simulink model "example6"  (Simulink 7.1)
settings: Solver=ode45  StartTime=0.0  StopTime=10.0  MaxStep=0.1  RelTol=1e-3
model workspace: external: M-Code (data not in the file)
undefined symbols (not defined in the file): doubleElbow, FDgq, J
libraries: simulink x5
settings Model: Creator=roy  LastModifiedBy=roy
settings DataIOCC: LimitDataPoints=off

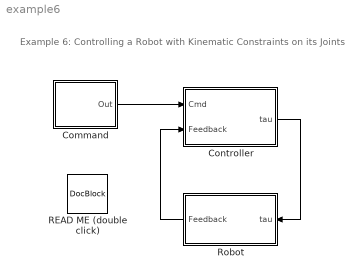
== system example6 ==
  note: Example 6: Controlling a Robot with
      | Kinematic Constraints on its Joints
  Command : Subsystem
  Controller : Subsystem
  READ ME (double click) : simulink/Model-Wide Utilities/DocBlock  SystemSampleTime=-1  DocumentType=Text
      content=|
      | This Simulink model follows on from Example 1 (with organizational
      | elements from Example 2), in which a simple PD control law was used to
      | control the motion of a planar 2R robot mechanism.  The new feature in
      | this example is that the robot is subject to a kinematic constraint on its
      | joint variables.
      |
      | Specifically, the robot in this example is a modification of the planar 2R
      | mechanism in which the elbow joint has been replaced by a pair of revolute
      | joints close together, which are subject to a 1:1 gearing constraint
      | (i.e., the two joint variables are constrained to be the same).  This is
      | the kind of joint one gets from two equal-radius cylinders rolling over
      | each other without slipping.  The robot therefore has three joint
      | variables in total, but q(2) is constrained to be equal to q(3).
      |
      | There is also a new feature to be found in the control system.  The
      | controller is interested in controlling this robot as if the elbow were a
      | single compound joint with a single joint variable.  Therefore, the
      | controller seeks to control the two variables q(1) and q(2)+q(3), the
      | latter being the angle between the two main links in the mechanism; and
      | the signal generated by the command subsystem consists of a commanded
      | value for q(1) and a commanded value for q(2)+q(3).  The controller
      | subsystem therefore contains extra blocks that translate from the
      | mechanism's joint space to the control system's command space and back
      | again.  For more details, see the controller subsystem's documantation
      | block.
      |
      | The dynamics calculation for a mechanism with kinematic constraints among
      | its joint variables is performed by FDgq.  This function expects to find a
      | field called "gamma_q" in the model data structure, containing the handle
      | of a function that formulates the constraint equations.  FDgq then solves
      | the equation of motion in a manner that complies with the constraints.
      | More details can be found in the documentation block in the robot
      | subsystem.
      |
      | If you run this simulation, then you will immediately see that the
      | controller is badly tuned, just like in Example 1, so you can see the
      | dynamics in action.  It is particularly obvious that the wobbling when the
      | robot is straight is at a lower frequency, and is less damped, than the
      | wobbling when the robot is bent.  Adjusting the gains (in particular,
      | higher gains for joint 1) will improve the performance.  In contrast to
      | the poor tracking accuracy of the control system, the kinematic constraint
      | on q(2) and q(3) is maintained exactly.
      |
      | To view the motion with showmotion, use the command
      | "showmotion(doubleElbow,tout,qout)".
  Robot : Subsystem  Orientation=left
  wires:
  Command/1(Out) -> Controller/1(Cmd)
  Robot/1(Feedback) -> Controller/2(Feedback)
  Controller/1(tau) -> Robot/1(tau)

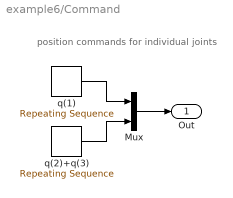
== system example6/Command ==
  note: position commands for
      | individual joints
  Mux : Mux  Inputs=2
  q(1) : simulink/Sources/Repeating Sequence  SystemSampleTime=-1  rep_seq_t=[0 1 2 3 4]  rep_seq_y=[0 1 1 0 0]
  q(2)+q(3) : simulink/Sources/Repeating Sequence  SystemSampleTime=-1  rep_seq_t=[0 1 2 3 4]  rep_seq_y=[0 2.5 2.5 0 0]
  Out : Outport  OutDataType=sfix(16)  OutScaling=2^0
  wires:
  q(1)/1 -> Mux/1
  q(2)+q(3)/1 -> Mux/2
  Mux/1 -> Out/1

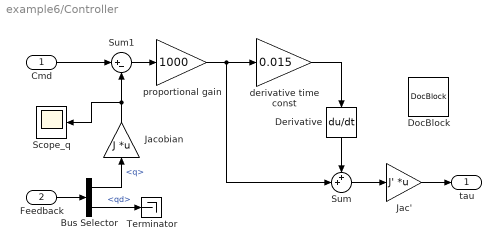
== system example6/Controller ==
  Cmd : Inport  OutDataType=sfix(16)  OutScaling=2^0
  Feedback : Inport  Port=2  OutDataType=sfix(16)  OutScaling=2^0
  Bus Selector : BusSelector  OutputSignals=q,qd
  Derivative : Derivative  Orientation=down
  DocBlock : simulink/Model-Wide Utilities/DocBlock  SystemSampleTime=-1  DocumentType=Text
      content=|
      | This subsystem implements a simple proportional-plus-derivative (PD)
      | controller resembling the one in Example 1.  The new feature in this
      | controller is a mismatch between the robot's joint space and the space in
      | which the controller operates.  The latter is often called "operational
      | space".
      |
      | The term "operational space" (or "task space") usually refers to the space
      | of Cartesian coordinates of the end-effector of an industrial robot arm.
      | Or, it may refer to the collection of coordinates that specify the
      | locations of a humanoid robot's hands, feet, head and centre of mass.  The
      | technique of controlling a robot directly in its operational space is
      | called "Operational-Space Control", and was pioneered by Khatib.
      |
      | In this example, we have an especially simple operational space.  If we
      | define it by means of two variables, x(1) and x(2), then x(1) = q(1) and
      | x(2) = q(2)+q(3) (=total bend angle at the elbow).  We can therefore
      | define a matrix, J, that maps q to x (i.e., x=J*q).  This matrix has the
      | value [1 0 0; 0 1 1], and is defined in the model workspace of this
      | Simulink model.  This matrix is the partial derivative of x with respect
      | to q, and is called the Jacobian.  In the general case, the Jacobian can
      | be used only to map the velocity variables.  However, in this particular
      | example, it works for the position variables too.
      |
      | The workings of the control system can now be explained as follows.
      | First, the incoming joint position signal, q, is converted to operational
      | space and subtracted from the command signal.  The difference (the
      | tracking error in operational space) is then fed into the blocks that
      | implement the PD control law; and then the result is converted back to
      | joint space by multiplying it by the transpose of the Jacobian.  The
      | reason we use the transpose here, rather than (e.g.) the pseudoinverse, is
      | that the signal at this point now represents a force to be applied to the
      | robot.  (One of the basic properties of Jacobians is that if J maps
      | velocities from space A to space B then J' maps forces from space B* to
      | space A*, where A* and B* are the force spaces associated with the
      | velocity spaces A and B, respectively.)
      |
      | One of the more subtle effects of a kinematic constraint on the joint
      | position variables is that they introduce redundancy into the force
      | variables.  In this example, because the constraint forces q(2)==q(3), we
      | find that only the sum of tau(2) and tau(3) matters.  Thus, for any force
      | f, applying tau(2)+f to joint 2 and tau(3)-f to joint 3 has the same
      | effect as applying tau(2) to joint 2 and tau(3) to joint 3.  This control
      | system has sent equal values to both joints (i.e., tau(2)==tau(3)), but it
      | could instead have sent 2*tau(2) to joint 2 and 0 to joint 3, or vice
      | versa -- it is an arbitrary choice.  (However, in practice you have to
      | apply the forces at the joints where the actuators are.)
      |
      | This control system, like the one in Example 1, is deliberately badly
      | tuned.  Better performance can be obtained by using different gains for
      | joint 1 and joint 2+3, and making the gains for joint 1 larger.  The gains
      | [3000;1000] and [0.06;0.02] will give better results.
  Jac' : Gain  Gain=J'  Multiplication=Matrix(K*u)  ParameterDataType=sfix(16)  ParameterScaling=2^0  OutDataType=sfix(16)  OutScaling=2^0
  Jacobian : Gain  Orientation=up  Gain=J  Multiplication=Matrix(K*u)  ParameterDataType=sfix(16)  ParameterScaling=2^0  OutDataType=sfix(16)  OutScaling=2^0
  Scope_q : Scope
      settings: YMin=-0.2  YMax=2.7
  Sum : Sum  Inputs=++|  OutDataType=sfix(16)  OutScaling=2^0
  Sum1 : Sum  Inputs=|+-  OutDataType=sfix(16)  OutScaling=2^0
  Terminator : Terminator
  derivative time const : Gain  Gain=0.015  ParameterDataType=sfix(16)  ParameterScaling=2^0  OutDataType=sfix(16)  OutScaling=2^0
  proportional gain : Gain  Gain=1000  ParameterDataType=sfix(16)  ParameterScaling=2^0  OutDataType=sfix(16)  OutScaling=2^0
  tau : Outport  OutDataType=sfix(16)  OutScaling=2^0
  wires:
  Sum1/1 -> proportional gain/1
  proportional gain/1 -> Sum/2, derivative time const/1
  Sum/1 -> Jac'/1
  Feedback/1 -> Bus Selector/1
  Bus Selector/2 -> Terminator/1  "<qd>"
  Cmd/1 -> Sum1/1
  Derivative/1 -> Sum/1
  derivative time const/1 -> Derivative/1
  Jac'/1 -> tau/1
  Bus Selector/1 -> Jacobian/1  "<q>"
  Jacobian/1 -> Sum1/2, Scope_q/1

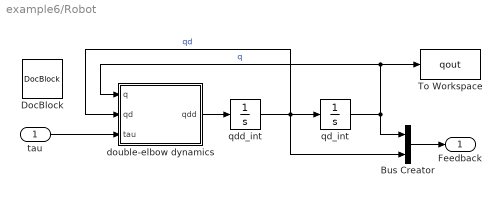
== system example6/Robot ==
  tau : Inport  OutDataType=sfix(16)  OutScaling=2^0
  Bus Creator : BusCreator  Inputs=2
  DocBlock : simulink/Model-Wide Utilities/DocBlock  SystemSampleTime=-1  DocumentType=Text
      content=|
      | This subsystem is responsible for calculating the dynamics of the robot.
      | It is essentially the same as the corresponding subsystem in Example 2.
      | The only significant difference is that the dynamics in this example is
      | being calculated by the function FDgq instead of FDab.
      |
      | The presence of kinematic constraints among the joint variables does not
      | significantly disturb the process of dynamics calculation.  The procedure
      | is essentially the same as for a mechanism without constraints: call a
      | dynamics function, integrate its output variable (qdd) twice to get qd and
      | q, and feed them back to the dynamics function.
      |
      | However, the presence of kinematic constraints can complicate the task of
      | setting correct initial conditions.  The problem is, of course, that one
      | must find initial values for q and qd that satisfy the constraints.  In
      | this particular example, the problem is trivial: the initial values are
      | zero.  However, in systems with more complicated constraints, it may be
      | necessary to calculate correct initial values.  One possibility is to do
      | this calculation at the time the model data structure is being created,
      | and store the result in fields with names like "q_init" and "qd_init".  If
      | you follow this route, then the Simulink model's workspace could be
      | initialized with Matlab code that includes the following lines:
      |
      |   model = modelcreatorfn( arguments... );
      |   q_init = model.q_init;
      |   qd_init = model.qd_init;
      |
      | Alternatively, if you can come up with a guess that's close, then you can
      | use the model's gamma_q function directly.  In this case, the Matlab code
      | is
      |
      |   model = modelcreatorfn( arguments... );
      |   q_init_guess = ....;
      |   qd_init_guess = ....;
      |   [q_init, qd_init] = model.gamma_q( q_init_guess, qd_init_guess );
      |
      | The reason why this second approach works is because one of the jobs of
      | gamma_q is to return values of q and qd that comply exactly with the
      | constraints (or, at the very least, comply more accurately than the values
      | in the argument list).
  To Workspace : ToWorkspace  VariableName=qout  SampleTime=-1  SaveFormat=Array
  double-elbow dynamics : Subsystem
  qd_int : Integrator
  qdd_int : Integrator
  Feedback : Outport  OutDataType=sfix(16)  OutScaling=2^0
  wires:
  Bus Creator/1 -> Feedback/1
  tau/1 -> double-elbow dynamics/3(tau)
  double-elbow dynamics/1(qdd) -> qdd_int/1
  qdd_int/1 -> qd_int/1, double-elbow dynamics/2(qd), Bus Creator/2  "qd"
  qd_int/1 -> Bus Creator/1, double-elbow dynamics/1(q), To Workspace/1  "q"

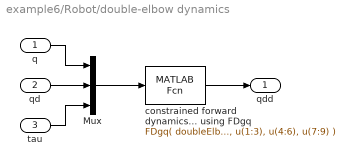
== system example6/Robot/double-elbow dynamics ==
  q : Inport  OutDataType=sfix(16)  OutScaling=2^0
  qd : Inport  Port=2  OutDataType=sfix(16)  OutScaling=2^0
  tau : Inport  Port=3  OutDataType=sfix(16)  OutScaling=2^0
  Mux : Mux  Inputs=3
  constrained forward dynamics using FDgq : MATLABFcn  MATLABFcn=FDgq( doubleElbow, u(1:3), u(4:6), u(7:9) )  OutputDimensions=[3 1]  OutputSignalType=real  Output1D=off
  qdd : Outport  OutDataType=sfix(16)  OutScaling=2^0
  wires:
  qd/1 -> Mux/2
  q/1 -> Mux/1
  tau/1 -> Mux/3
  Mux/1 -> constrained forward dynamics using FDgq/1
  constrained forward dynamics using FDgq/1 -> qdd/1
